simulink model "TurtlebotSim"  (R2021b)
settings: Solver=ode4  StartTime=0.0  StopTime=10.0  FixedStep=0.01  RelTol=1e-3
values from neighbouring files (symbols this model uses):
  x0 = [0;0;0]    [config.m]
settings Model: Creator=delur  LastModifiedBy=delur

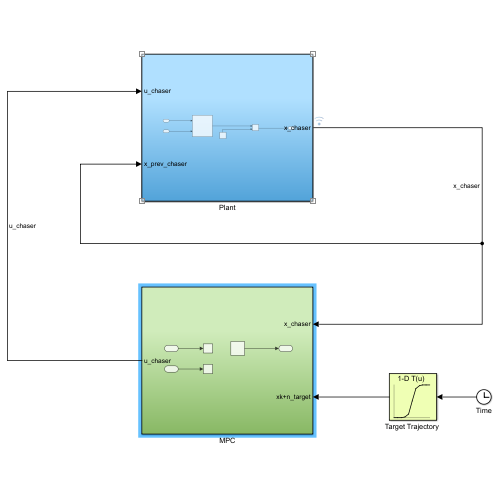
[thumbnail: Simulink's stored preview of the top-level diagram]
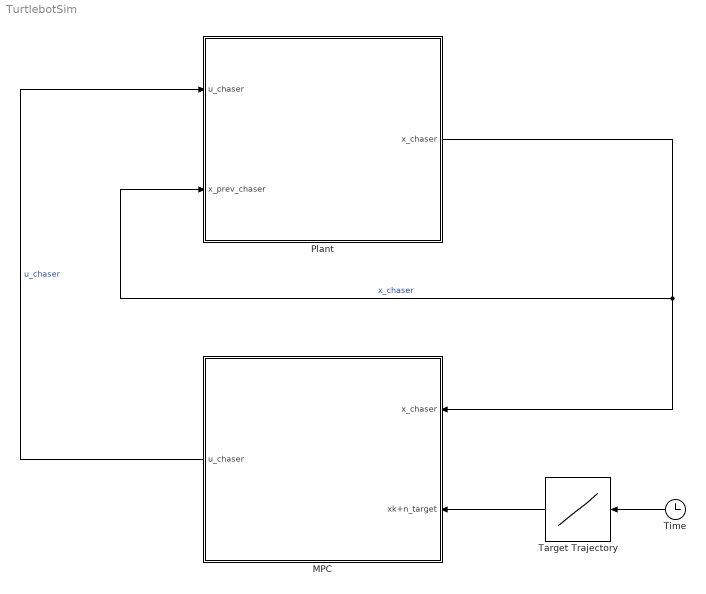
== system TurtlebotSim ==
  MPC : Subsystem
  Plant : Subsystem
  "Target Trajectory " : Lookup_n-D  NumberOfTableDimensions=1  BreakpointsForDimension1=[-5:5]  Table=tanh([-5:5])  InternalRulePriority=Speed  RndMeth=Simplest  InputSameDT=on
  Time : Clock
  wires:
  Plant/1(x_chaser) -> Plant/2(x_prev_chaser), MPC/1(x_chaser)  "x_chaser"
  MPC/1(u_chaser) -> Plant/1(u_chaser)  "u_chaser"
  "Target Trajectory "/1 -> MPC/2(xk+n_target)
  Time/1 -> "Target Trajectory "/1

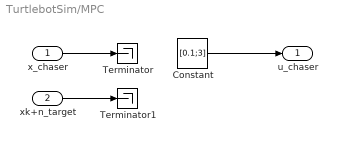
== system TurtlebotSim/MPC ==
  x_chaser : Inport
  xk+n_target : Inport  Port=2
  Constant : Constant  Value=[0.1;3]
  Terminator : Terminator
  Terminator1 : Terminator
  u_chaser : Outport
  wires:
  x_chaser/1 -> Terminator/1
  xk+n_target/1 -> Terminator1/1
  Constant/1 -> u_chaser/1

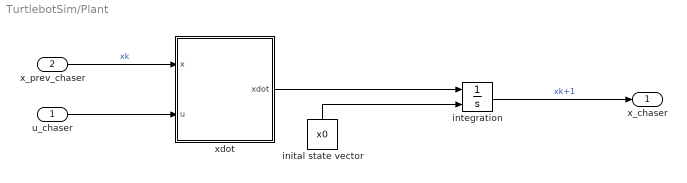
== system TurtlebotSim/Plant ==
  u_chaser : Inport
  x_prev_chaser : Inport  Port=2
  inital state vector : Constant  Value=x0
  integration : Integrator  InitialConditionSource=external
  xdot : MATLAB Function  TreatAsAtomicUnit=on
  x_chaser : Outport
  wires:
  u_chaser/1 -> xdot/2(u)
  integration/1 -> x_chaser/1  "xk+1"
  x_prev_chaser/1 -> xdot/1(x)  "xk"
  xdot/1(xdot) -> integration/1
  inital state vector/1 -> integration/2

== matlab function TurtlebotSim/Plant/xdot ==
  data: x input; u input; xdot output
function xdot = dynamics(x,u)
% STATE VECTOR X: [theta,x,y], [orientation, x pos inertial, y pos inertial
% (pose state)
% CONTROL INPUT u: [uw,uv], [angular rate, linear velocity] (twist control)
xdot = zeros(3,1);

xdot(1) = u(1); % theta_dot
xdot(2) = u(2)*cos(x(1)); %x inertial velocity
xdot(3) = u(2)*sin(x(1)); %y inertial velocity

end
